simulink model "lclowpass_4"  (R2016b)
settings: Solver=ode15s  StartTime=0.0  StopTime=1  RelTol=1e-3
values from neighbouring files (symbols this model uses):
  C = 0.0047    [rlcsolver.m]
  L = 1e-10    [rlcsolver.m]
  Ln = 1e-10    [rlcsolver.m]
  PerT = 0.1    [rlcsolver.m]
  PerV = 6    [rlcsolver.m]
  R = 146    [rlcsolver.m]
  Rn = 4.4    [rlcsolver.m]
settings Model: Creator=Brian  LastModifiedBy=Brian

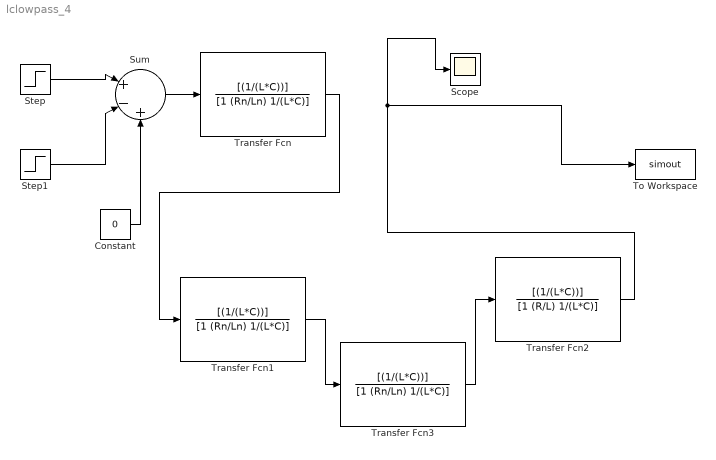
== system lclowpass_4 ==
  Constant : Constant  Value=0
  Scope : Scope
  Step : Step  Time=0  After=PerV  SampleTime=0
  Step1 : Step  Time=PerT  After=PerV  SampleTime=0
  Sum : Sum  Inputs=|+-+
  To Workspace : ToWorkspace  VariableName=simout  SaveFormat=Timeseries  SampleTime=-1
  Transfer Fcn : TransferFcn  Numerator=[(1/(L*C))]  Denominator=[1 (Rn/Ln) 1/(L*C)]
  Transfer Fcn1 : TransferFcn  Numerator=[(1/(L*C))]  Denominator=[1 (Rn/Ln) 1/(L*C)]
  Transfer Fcn2 : TransferFcn  Numerator=[(1/(L*C))]  Denominator=[1 (R/L) 1/(L*C)]
  Transfer Fcn3 : TransferFcn  Numerator=[(1/(L*C))]  Denominator=[1 (Rn/Ln) 1/(L*C)]
  wires:
  Transfer Fcn2/1 -> To Workspace/1, Scope/1
  Sum/1 -> Transfer Fcn/1
  Step/1 -> Sum/1
  Step1/1 -> Sum/2
  Constant/1 -> Sum/3
  Transfer Fcn/1 -> Transfer Fcn1/1
  Transfer Fcn1/1 -> Transfer Fcn3/1
  Transfer Fcn3/1 -> Transfer Fcn2/1
